simulink model "ysw2_6"  (R2014a)
settings: Solver=ode45  StartTime=0.0  StopTime=10.0  RelTol=1e-3
settings Model: Creator=Administrator  LastModifiedBy=Administrator

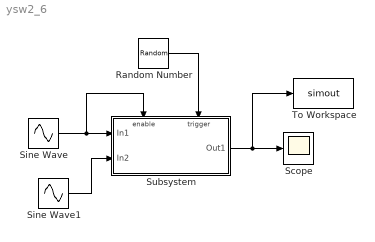
== system ysw2_6 ==
  Random Number : RandomNumber  SampleTime=0.1
  Scope : Scope
  Sine Wave : Sin  Amplitude=3  SampleTime=0
  Sine Wave1 : Sin  SampleTime=0
  Subsystem : Subsystem
  To Workspace : ToWorkspace  VariableName=simout  SampleTime=-1
  wires:
  Sine Wave1/1 -> Subsystem/2(In2)
  Subsystem/1(Out1) -> To Workspace/1, Scope/1
  Sine Wave/1 -> Subsystem/Enable, Subsystem/1(In1)
  Random Number/1 -> Subsystem/Trigger

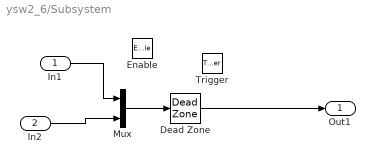
== system ysw2_6/Subsystem ==
  In1 : Inport
  In2 : Inport  Port=2
  Enable : EnablePort
  Trigger : TriggerPort  PortDimensions=1
  Dead Zone : DeadZone  SaturateOnIntegerOverflow=on
  Mux : Mux  Inputs=2
  Out1 : Outport
  wires:
  In1/1 -> Mux/1
  Mux/1 -> Dead Zone/1
  Dead Zone/1 -> Out1/1
  In2/1 -> Mux/2
